simulink model "Simulation_04"  (R2014a)
settings: Solver=ode45  StartTime=0.0  StopTime=10.0  RelTol=1e-3
undefined symbols (not defined in the file or in its folder): sigbuilder_block
libraries: powerlib x12, simulink x1, powerlib_meascontrol x1
settings Model: Creator=Dell  LastModifiedBy=Dell

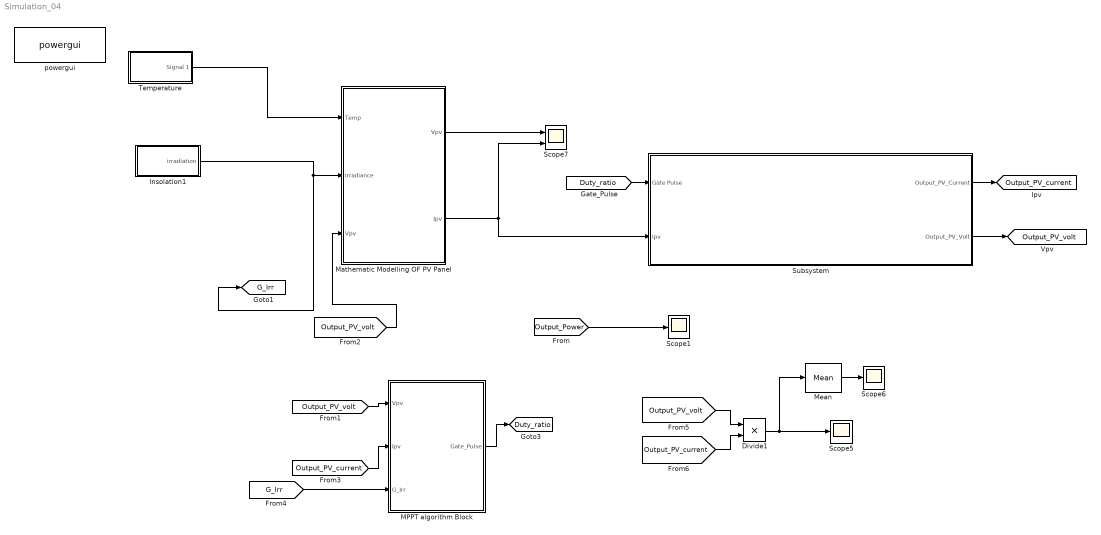
== system Simulation_04 ==
  Divide1 : Product  Inputs=**
  Insolation1 : Subsystem  Tag=STV Subsys  LoadFcn=sigbuilder_block('load');  StartFcn=sigbuilder_block('start');  StopFcn=sigbuilder_block('stop');  ClipboardFcn=sigbuilder_block('clipboard');  mask(Sigbuilder block){}
      mask help: Simulink:masks:SigbuilderBlock_MD
      mask init:
      | if ~strcmp(get_param(bdroot(gcbh),'SimulationStatus'),'stopped') tuvar = sigbuilder_block('maskInit'); end
      settings: CopyFcn=sigbuilder_block('copy');  DeleteFcn=sigbuilder_block('delete');  ModelCloseFcn=sigbuilder_block('modelClose');  PreSaveFcn=sigbuilder_block('preSave');  PauseFcn=sigbuilder_block('pause')  ContinueFcn=sigbuilder_block('continue')  NameChangeFcn=sigbuilder_block('namechange');  OpenFcn=sigbuilder_block('open',[557.25 17.25 550.5 394.5 ]);  CloseFcn=sigbuilder_block('close');
      mask Display: plot(0, 0, 100, 100,[2, 2, 32, 32, 2], [68, 8, 8, 68, 68],[32, 2], [38, 38], [32, 19, 2],[53, 60, 44], [32, 17, 17, 2],[16, 16, 31, 31]);txt = getActiveGroup(gcbh);text(2, 100, txt,'verticalAlignment', 'top');
  MPPT algorithm Block : Subsystem
  Mathematic Modelling OF PV Panel : Subsystem
      mask Display:
      | plot([0.3 0.4],[0.4 0.8]);
      | plot([0.4 0.5],[0.4 0.8]);
      | plot([0.5 0.6],[0.4 0.8]);
      | plot([0.6 0.7],[0.4 0.8]);
      | plot([0.3 0.6],[0.4 0.4]);
      | plot([0.325 0.625],[0.5 0.5]);
      | plot([0.35 0.65],[0.6 0.6]);
      | plot([0.375 0.675],[0.7 0.7]);
      | plot([0.4 0.7],[0.8 0.8]);
      | text(0.52,0.75,'PV module (V)','horizontalAlignment', 'center');
  Mean : powerlib_meascontrol/Measurements/Mean  Freq=60  Vinit=0  Ts=0
  Scope1 : Scope
      settings: TimeRange=2  YMin=220  YMax=252.5  SaveName=ScopeData2
  Scope5 : Scope
      settings: TimeRange=0.8  YMin=222.5  YMax=262.5  SaveName=ScopeData6
  Scope6 : Scope
      settings: TimeRange=0.8  YMin=258.52  YMax=258.65  SaveName=ScopeData7
  Scope7 : Scope  NumInputPorts=2
      settings: YMin=-22.5~7.325  YMax=35~7.6
  Subsystem : Subsystem
  Temperature : Subsystem  Tag=STV Subsys  LoadFcn=sigbuilder_block('load');  StartFcn=sigbuilder_block('start');  StopFcn=sigbuilder_block('stop');  ClipboardFcn=sigbuilder_block('clipboard');  mask(Sigbuilder block){}
      mask help: Simulink:masks:SigbuilderBlock_MD
      mask init:
      | if ~strcmp(get_param(bdroot(gcbh),'SimulationStatus'),'stopped') tuvar = sigbuilder_block('maskInit'); end
      settings: CopyFcn=sigbuilder_block('copy');  DeleteFcn=sigbuilder_block('delete');  ModelCloseFcn=sigbuilder_block('modelClose');  PreSaveFcn=sigbuilder_block('preSave');  PauseFcn=sigbuilder_block('pause');  ContinueFcn=sigbuilder_block('continue');  NameChangeFcn=sigbuilder_block('namechange');  OpenFcn=sigbuilder_block('open',[437.25 180 550.5 395.25 ]);  CloseFcn=sigbuilder_block('close');
      mask Display: plot(0, 0, 100, 100,[2, 2, 32, 32, 2], [68, 8, 8, 68, 68],[32, 2], [38, 38], [32, 19, 2],[53, 60, 44], [32, 17, 17, 2],[16, 16, 31, 31]);txt = getActiveGroup(gcbh);text(2, 100, txt,'verticalAlignment', 'top');
  powergui : powerlib/powergui  Priority=1  SimulationMode=Discrete  SolverType=Tustin  SampleTime=1e-6  frequency=60  SPID=off  DisableSnubberDevices=off  DisableRonSwitches=off  DisableVfSwitches=off  SwTol=0  Interpol=off  DisplayEquations=off  Ts=0  methode=off  frequencyindice=0  Pbase=100e6  ErrMax=1e-4  Iterations=50  UnitsV=kV  UnitsW=MW  FunctionMessages=off  echomessages=off  HookPort=off  EnableUseOfTLC=off  x0status=blocks  RestoreLinks=warning  ResistiveCurrentMeasurement=off  Frange=[0:2:500]  Ylog=off  Xlog=on  ShowGrid=off  save=off  variable=ZData  structure=0  ZoomFFT=off  StartTime=0.0  cycles=1  DisplayStyle=1  fundamental=60  FreqAxis=off  MaxFrequency=1000  frequencyindicesteady=1  RmsSteady=1  display=off
  tag scope: Duty_ratio=global, G_Irr=global, Output_PV_current=global, Output_PV_volt=global
  wires:
  [Output_Power] -> Scope1/1
  [Output_PV_volt] -> Divide1/1
  [Output_PV_current] -> Divide1/2
  Divide1/1 -> Scope5/1, Mean/1
  Mean/1 -> Scope6/1
  Temperature/1(Signal 1) -> Mathematic Modelling OF PV Panel/1(Temp)
  Insolation1/1(irradiation) -> [G_Irr], Mathematic Modelling OF PV Panel/2(Irradiance)
  Mathematic Modelling OF PV Panel/2(Ipv) -> Subsystem/2(Ipv), Scope7/2
  [Output_PV_volt] -> Mathematic Modelling OF PV Panel/3(Vpv)
  [Duty_ratio] -> Subsystem/1(Gate Pulse)
  Subsystem/1(Output_PV_Current) -> [Output_PV_current]
  Subsystem/2(Output_PV_Volt) -> [Output_PV_volt]
  [Output_PV_volt] -> MPPT algorithm Block/1(Vpv)
  [Output_PV_current] -> MPPT algorithm Block/2(Ipv)
  MPPT algorithm Block/1("Gate_Pulse ") -> [Duty_ratio]
  Mathematic Modelling OF PV Panel/1("Vpv ") -> Scope7/1
  [G_Irr] -> MPPT algorithm Block/3(G_Irr)

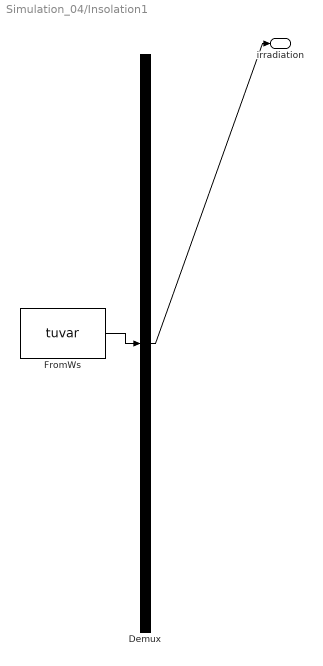
== system Simulation_04/Insolation1 ==
  Demux : Demux  Tag=STV Demux  Outputs=1
  FromWs : FromWorkspace  Tag=STV FromWs  VariableName=tuvar  SampleTime=0
      SigBuilderData=|
      | common.afterFinalStr = 'Extrapolate'
      | common.sampleTime = 0
      | dataSet.timeRange = [0 6]
      | dataSet.name = 'Group 1'
      | sbobj.Groups.Name = 'Group 1'
      | sbobj.Groups.Signals.Name = 'irradiation'
      | sbobj.Groups.Signals.XData = [0 2 3.99 4 6]
      | sbobj.Groups.Signals.YData = [1 1 1 1 1]
  irradiation : Outport  Tag=STV Outport
  wires:
  FromWs/1 -> Demux/1
  Demux/1 -> irradiation/1

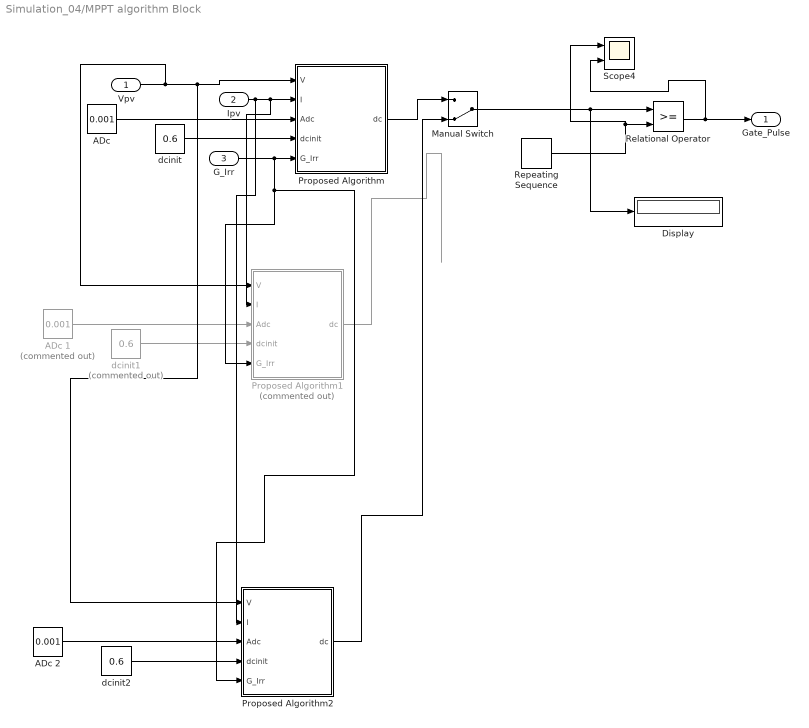
== system Simulation_04/MPPT algorithm Block ==
  Vpv : Inport
  Ipv : Inport  Port=2
  G_Irr : Inport  Port=3
  "ADc\t" : Constant  Value=0.001
  ADc	1 : Constant  Commented=on  Value=0.001
  ADc	2 : Constant  Value=0.001
  Display : Display
  Manual Switch : ManualSwitch  CurrentSetting=0
  Proposed Algorithm : MATLAB Function  TreatAsAtomicUnit=on
  Proposed Algorithm1 : MATLAB Function  Commented=on  TreatAsAtomicUnit=on
  Proposed Algorithm2 : MATLAB Function  TreatAsAtomicUnit=on
  Relational Operator : RelationalOperator  OutDataTypeStr=boolean
  Repeating Sequence : simulink/Sources/Repeating Sequence  rep_seq_t=[0 1/40000 1/20000]  rep_seq_y=[0 1 0]
  Scope4 : Scope  NumInputPorts=2
      settings: YMin=0~0  YMax=1~1  SaveName=ScopeData5
  dcinit : Constant  Value=0.6
  dcinit1 : Constant  Commented=on  Value=0.6
  dcinit2 : Constant  Value=0.6
  "Gate_Pulse " : Outport
  wires:
  Relational Operator/1 -> "Gate_Pulse "/1, Scope4/2
  Repeating Sequence/1 -> Scope4/1, Relational Operator/2
  dcinit/1 -> Proposed Algorithm/4(dcinit)
  "ADc\t"/1 -> Proposed Algorithm/3(Adc)
  dcinit1/1 -> Proposed Algorithm1/4(dcinit)
  ADc	1/1 -> Proposed Algorithm1/3(Adc)
  Proposed Algorithm/1(dc) -> Manual Switch/1
  Proposed Algorithm1/1(dc) -> ?
  Manual Switch/1 -> Display/1, Relational Operator/1
  Ipv/1 -> Proposed Algorithm2/2(I), Proposed Algorithm1/2(I), Proposed Algorithm/2(I)
  Vpv/1 -> Proposed Algorithm2/1(V), Proposed Algorithm/1(V), Proposed Algorithm1/1(V)
  dcinit2/1 -> Proposed Algorithm2/4(dcinit)
  ADc	2/1 -> Proposed Algorithm2/3(Adc)
  G_Irr/1 -> Proposed Algorithm2/5(G_Irr), Proposed Algorithm1/5(G_Irr), Proposed Algorithm/5(G_Irr)
  Proposed Algorithm2/1(dc) -> Manual Switch/2

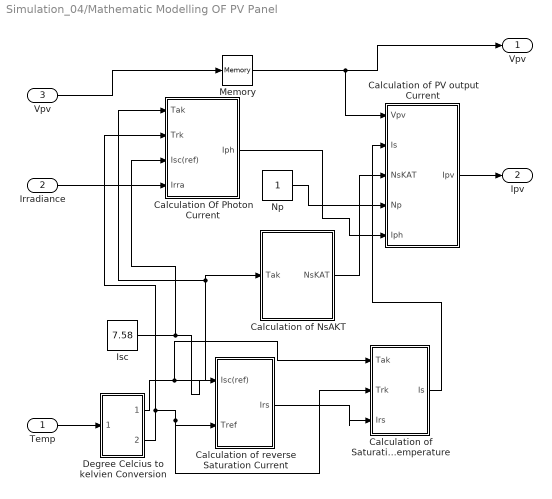
== system Simulation_04/Mathematic Modelling OF PV Panel ==
  Temp : Inport
  Irradiance : Inport  Port=2
  Vpv : Inport  Port=3
  "Calculation Of Photon Current " : Subsystem
  Calculation of Saturation Current Varies With Temperature : Subsystem
  Calculation of NsAKT : Subsystem
  "Calculation of PV output Current " : Subsystem
  Calculation of reverse Saturation Current : Subsystem
  Degree Celcius to kelvien Conversion : Subsystem
  Isc : Constant  Value=7.58
  Memory : Memory
  Np : Constant
  "Vpv " : Outport
  Ipv : Outport  Port=2
  wires:
  Calculation of Saturation Current Varies With Temperature/1(Is) -> "Calculation of PV output Current "/2(Is)
  Calculation of reverse Saturation Current/1(Irs) -> Calculation of Saturation Current Varies With Temperature/3("Irs ")
  Np/1 -> "Calculation of PV output Current "/4(Np)
  Temp/1 -> Degree Celcius to kelvien Conversion/1("Top ")
  "Calculation of PV output Current "/1("Ipv ") -> Ipv/1
  Irradiance/1 -> "Calculation Of Photon Current "/4(Irra)
  Degree Celcius to kelvien Conversion/1(Tak) -> Calculation of Saturation Current Varies With Temperature/1(Tak), "Calculation Of Photon Current "/1(Tak), Calculation of NsAKT/1("Tak ")
  "Calculation Of Photon Current "/1(Iph) -> "Calculation of PV output Current "/5(Iph)
  Calculation of NsAKT/1(NsKAT) -> "Calculation of PV output Current "/3(NsKAT)
  Isc/1 -> "Calculation Of Photon Current "/3(Isc(ref)), Calculation of reverse Saturation Current/1("Isc(ref) ")
  Degree Celcius to kelvien Conversion/2(Trk) -> "Calculation Of Photon Current "/2(Trk), Calculation of Saturation Current Varies With Temperature/2("Trk "), Calculation of reverse Saturation Current/2("Tref ")
  Vpv/1 -> Memory/1
  Memory/1 -> "Calculation of PV output Current "/1(Vpv), "Vpv "/1

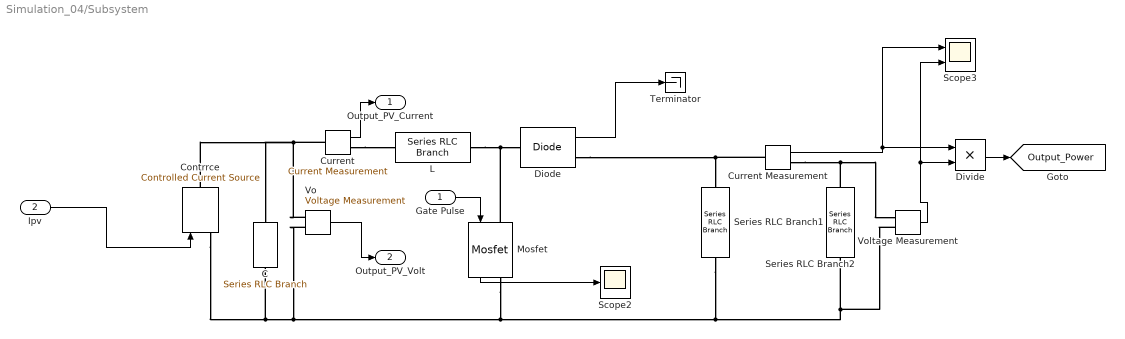
== system Simulation_04/Subsystem ==
  Gate Pulse : Inport
  Ipv : Inport  Port=2
  C : powerlib/Elements/Series RLC Branch  LConnTagsString=__new0  RConnTagsString=__new0  BranchType=C  Resistance=10  Inductance=5e-3  SetiL0=on  InitialCurrent=0  Capacitance=1e-6  Setx0=off  InitialVoltage=0  Measurements=None
  Contrrce : powerlib/Electrical Sources/Controlled Current Source  Initialize=on  Source_Type=DC  Amplitude=0  Phase=0  Frequency=0  Measurements=None
  "Current " : powerlib/Measurements/Current Measurement  PhasorSimulation=off  OutputType=Complex  PSBequivalent=0
  Current Measurement : powerlib/Measurements/Current Measurement  PhasorSimulation=off  OutputType=Complex  PSBequivalent=0
  Diode : powerlib/Power Electronics/Diode  Ron=0.001  Lon=0  Vf=0.8  IC=0  UseSnubber=off  Rs=500*0  Cs=250e-9*0  Measurements=on
  Divide : Product  Inputs=**
  L : powerlib/Elements/Series RLC Branch  LConnTagsString=__new0  RConnTagsString=__new0  BranchType=L  Resistance=10  Inductance=5e-3  SetiL0=on  InitialCurrent=0  Capacitance=1e-6  Setx0=off  InitialVoltage=0  Measurements=None
  Mosfet : powerlib/Power Electronics/Mosfet  Ron=0.1  Lon=0  Rd=0.01  Vfd=0  IC=0  Rs=1e5  Cs=inf  Measurements=on
  Scope2 : Scope
      settings: YMin=-5.49725  YMax=49.47525  SaveName=ScopeData3
  Scope3 : Scope  NumInputPorts=2
      settings: YMin=2.52~100.8  YMax=2.536~101.45  SaveName=ScopeData4
  Series RLC Branch1 : powerlib/Elements/Series RLC Branch  LConnTagsString=__new0  RConnTagsString=__new0  BranchType=C  Resistance=1  Inductance=5e-3  SetiL0=on  InitialCurrent=0  Capacitance=270e-6  Setx0=on  InitialVoltage=0  Measurements=None
  Series RLC Branch2 : powerlib/Elements/Series RLC Branch  LConnTagsString=__new0  RConnTagsString=__new0  BranchType=R  Resistance=60  Inductance=5e-3  SetiL0=on  InitialCurrent=0  Capacitance=1e-6  Setx0=off  InitialVoltage=0  Measurements=None
  Terminator : Terminator
  Vo : powerlib/Measurements/Voltage Measurement  PhasorSimulation=off  OutputType=Complex  PSBequivalent=0
  Voltage Measurement : powerlib/Measurements/Voltage Measurement  PhasorSimulation=off  OutputType=Complex  PSBequivalent=0
  Output_PV_Current : Outport
  Output_PV_Volt : Outport  Port=2
  tag scope: Output_Power=global
  wires:
  Ipv/1 -> Contrrce/1
  Diode/1 -> Terminator/1
  Divide/1 -> [Output_Power]
  Voltage Measurement/1 -> Scope3/2, Divide/2
  Vo/1 -> Output_PV_Volt/1
  Gate Pulse/1 -> Mosfet/1
  "Current "/1 -> Output_PV_Current/1
  Current Measurement/1 -> Divide/1, Scope3/1
  Mosfet/1 -> Scope2/1
  connections:
  Diode/RConn1 -- Current Measurement/LConn1 -- Series RLC Branch1/LConn1
  Vo/LConn1 -- Contrrce/RConn1 -- C/LConn1 -- "Current "/LConn1
  Series RLC Branch2/LConn1 -- Current Measurement/RConn1 -- Voltage Measurement/LConn1
  Contrrce/LConn1 -- C/RConn1 -- Vo/LConn2 -- Mosfet/RConn1 -- Series RLC Branch1/RConn1 -- Voltage Measurement/LConn2 -- Series RLC Branch2/RConn1
  "Current "/RConn1 -- L/LConn1
  L/RConn1 -- Mosfet/LConn1 -- Diode/LConn1

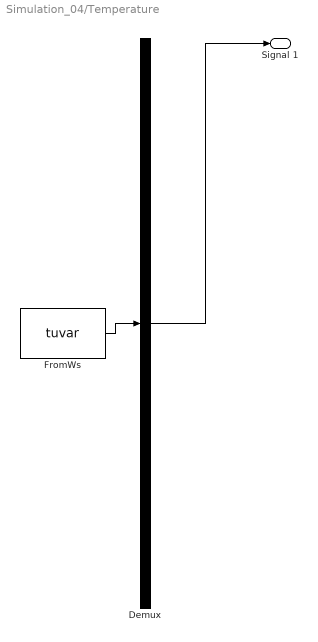
== system Simulation_04/Temperature ==
  Demux : Demux  Tag=STV Demux  Outputs=1
  FromWs : FromWorkspace  Tag=STV FromWs  VariableName=tuvar  SampleTime=0
      SigBuilderData=|
      | common.afterFinalStr = 'Extrapolate'
      | common.sampleTime = 0
      | dataSet.timeRange = [0 10]
      | dataSet.name = 'Group 1'
      | sbobj.Groups.Name = 'Group 1'
      | sbobj.Groups.Signals.Name = 'Signal 1'
      | sbobj.Groups.Signals.XData = [0 2 4 10]
      | sbobj.Groups.Signals.YData = [25 25 25 25]
  Signal 1 : Outport  Tag=STV Outport
  wires:
  Demux/1 -> Signal 1/1
  FromWs/1 -> Demux/1

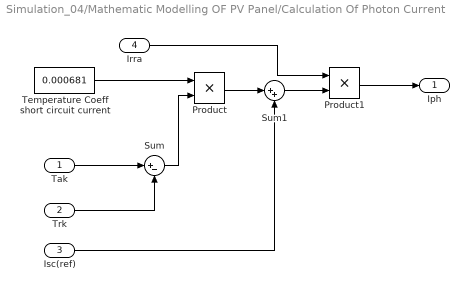
== system Simulation_04/Mathematic Modelling OF PV Panel/Calculation Of Photon Current  ==
  Tak : Inport
  Trk : Inport  Port=2
  Isc(ref) : Inport  Port=3
  Irra : Inport  Port=4
  Product : Product
  Product1 : Product
  Sum : Sum  Inputs=|+-
  Sum1 : Sum  Inputs=|++
  "Temperature Coeff short circuit current " : Constant  Value=0.000681
  Iph : Outport
  wires:
  Product/1 -> Sum1/1
  Trk/1 -> Sum/2
  "Temperature Coeff short circuit current "/1 -> Product/1
  Irra/1 -> Product1/1
  Isc(ref)/1 -> Sum1/2
  Tak/1 -> Sum/1
  Sum1/1 -> Product1/2
  Sum/1 -> Product/2
  Product1/1 -> Iph/1

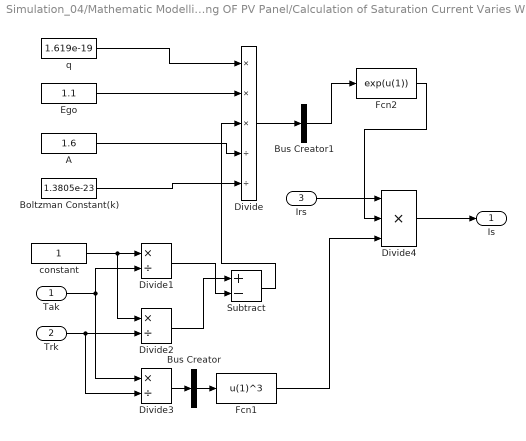
== system Simulation_04/Mathematic Modelling OF PV Panel/Calculation of Saturation Current Varies With Temperature ==
  Tak : Inport
  "Trk " : Inport  Port=2
  "Irs " : Inport  Port=3
  "A " : Constant  Value=1.6
  Boltzman Constant(k) : Constant  Value=1.3805e-23
  Bus Creator : BusCreator  Inputs=1
  Bus Creator1 : BusCreator  Inputs=1
  Divide : Product  Inputs=***//
  Divide1 : Product  Inputs=*/
  Divide2 : Product  Inputs=*/
  Divide3 : Product  Inputs=*/
  Divide4 : Product  Inputs=***
  Ego : Constant  Value=1.1
  Fcn1 : Fcn  Expr=u(1)^3
  Fcn2 : Fcn  Expr=exp(u(1))
  Subtract : Sum  Inputs=+-
  "constant " : Constant
  "q " : Constant  Value=1.619e-19
  Is : Outport
  wires:
  "constant "/1 -> Divide2/1, Divide1/1
  Bus Creator1/1 -> Fcn2/1
  Divide/1 -> Bus Creator1/1
  Divide1/1 -> Subtract/2
  Fcn1/1 -> Divide4/3
  Divide2/1 -> Subtract/1
  Tak/1 -> Divide1/2, Divide3/1
  Fcn2/1 -> Divide4/2
  "Trk "/1 -> Divide3/2, Divide2/2
  "A "/1 -> Divide/4
  Ego/1 -> Divide/2
  Subtract/1 -> Divide/3
  Boltzman Constant(k)/1 -> Divide/5
  "q "/1 -> Divide/1
  "Irs "/1 -> Divide4/1
  Divide4/1 -> Is/1
  Bus Creator/1 -> Fcn1/1
  Divide3/1 -> Bus Creator/1

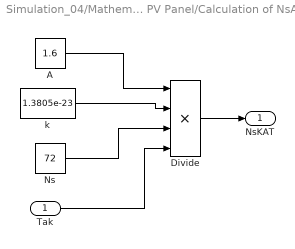
== system Simulation_04/Mathematic Modelling OF PV Panel/Calculation of NsAKT ==
  "Tak " : Inport
  A : Constant  Value=1.6
  Divide : Product  Inputs=****
  Ns : Constant  Value=72
  k : Constant  Value=1.3805e-23
  NsKAT : Outport
  wires:
  Ns/1 -> Divide/3
  A/1 -> Divide/1
  k/1 -> Divide/2
  "Tak "/1 -> Divide/4
  Divide/1 -> NsKAT/1

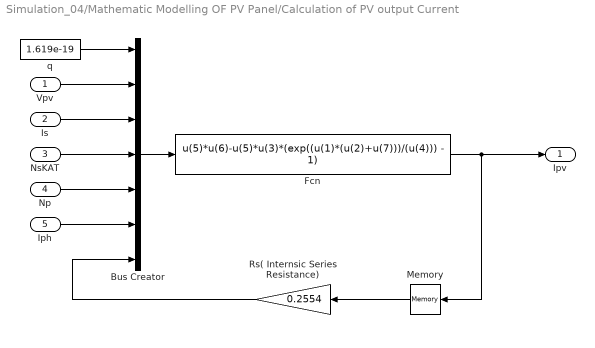
== system Simulation_04/Mathematic Modelling OF PV Panel/Calculation of PV output Current  ==
  Vpv : Inport
  Is : Inport  Port=2
  NsKAT : Inport  Port=3
  Np : Inport  Port=4
  Iph : Inport  Port=5
  Bus Creator : BusCreator  Inputs=7
  Fcn : Fcn  Expr=u(5)*u(6)-u(5)*u(3)*(exp((u(1)*(u(2)+u(7)))/(u(4))) - 1)
  Memory : Memory
  Rs( Internsic Series Resistance) : Gain  Gain=0.2554
  q : Constant  Value=1.619e-19
  "Ipv " : Outport
  wires:
  Vpv/1 -> Bus Creator/2
  Is/1 -> Bus Creator/3
  Fcn/1 -> Memory/1, "Ipv "/1
  Bus Creator/1 -> Fcn/1
  Rs( Internsic Series Resistance)/1 -> Bus Creator/7
  Iph/1 -> Bus Creator/6
  Np/1 -> Bus Creator/5
  q/1 -> Bus Creator/1
  NsKAT/1 -> Bus Creator/4
  Memory/1 -> Rs( Internsic Series Resistance)/1

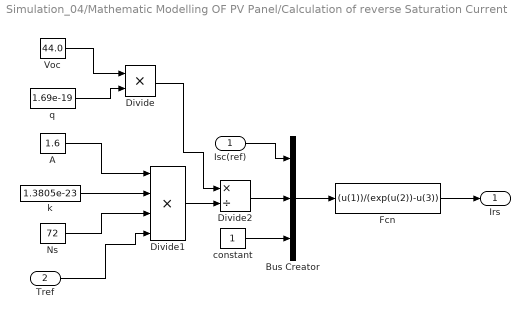
== system Simulation_04/Mathematic Modelling OF PV Panel/Calculation of reverse Saturation Current ==
  "Isc(ref) " : Inport
  "Tref " : Inport  Port=2
  A : Constant  Value=1.6
  Bus Creator : BusCreator  Inputs=3
  Divide : Product  Inputs=**
  Divide1 : Product  Inputs=****
  Divide2 : Product  Inputs=*/
  Fcn : Fcn  Expr=(u(1))/(exp(u(2))-u(3))
  Ns : Constant  Value=72
  Voc : Constant  Value=44.0
  "constant " : Constant
  k : Constant  Value=1.3805e-23
  q : Constant  Value=1.69e-19
  Irs : Outport
  wires:
  Voc/1 -> Divide/1
  Divide/1 -> Divide2/1
  k/1 -> Divide1/2
  "constant "/1 -> Bus Creator/3
  Divide2/1 -> Bus Creator/2
  Bus Creator/1 -> Fcn/1
  "Tref "/1 -> Divide1/4
  Fcn/1 -> Irs/1
  q/1 -> Divide/2
  A/1 -> Divide1/1
  "Isc(ref) "/1 -> Bus Creator/1
  Ns/1 -> Divide1/3
  Divide1/1 -> Divide2/2

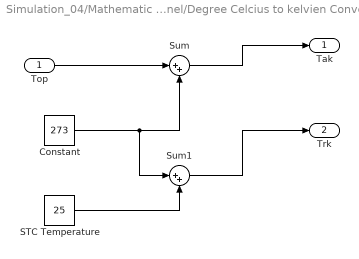
== system Simulation_04/Mathematic Modelling OF PV Panel/Degree Celcius to kelvien Conversion ==
  "Top " : Inport
  Constant : Constant  Value=273
  STC Temperature : Constant  Value=25
  Sum : Sum  Inputs=|++
  Sum1 : Sum  Inputs=|++
  Tak : Outport
  Trk : Outport  Port=2
  wires:
  Sum1/1 -> Trk/1
  Constant/1 -> Sum1/1, Sum/2
  "Top "/1 -> Sum/1
  Sum/1 -> Tak/1
  STC Temperature/1 -> Sum1/2

== matlab function Simulation_04/MPPT algorithm Block/Proposed Algorithm1 ==
  data: V input; dc output; I input; Adc input; dcinit input; G_Irr input
function dc = IC( V, I, Adc, dcinit, G_Irr)

 
% persistent dco Vo Io
% dataType = 'double';
%    
%             if isempty(Vo)
%                 Vo=0;
%                 Io=0;
%                 dco=dcinit;
%             end
% 
%           
%             dV=V-Vo;
%             dI=I-Io;
%           
%             if dV==0
%                 if dI==0
%                     dc =dco;
%                     return
%                 else
%                     if dI>0
%                         dc = dco + Adc; 
%                     else
%                         dc = dco - Adc; 
%                     end
%                 end
%             else
%                 if I+(dI/dV)*V==0
%                     dc=dco;
%                     return
%                 else
%                     if I+(dI/dV)*V>0
%                         dc = dco - Adc; 
%                     else
%                         dc = dco + Adc; 
%                     end
%                 end
%             end
%             dcmax=0.95; 
%               dcmin=0.05;
%             if dc>=dcmax || dc<=dcmin
%                 dc=dco;
%             end
% 
%             dco=dc;
%             Vo=V;
%             Io=I;
%      
persistent dmp Vo Io
dataType = 'double';
        
            if isempty(Vo)
             dmp=0.711;
             Vo=zeros(3,1);
             Io=zeros(3,1);
            end
            
            dc=dmp;
            Vo(1)=36.2;
            Io(1)=7.1;
            
          for i=2:3  
            if dc==0.69
                 dc=dmp -0.2*dmp;
                 Vo(i)=V;
                 Io(i)=I;
                 

 
 
  
     end

== matlab function Simulation_04/MPPT algorithm Block/Proposed Algorithm2 ==
  data: V input; dc output; I input; Adc input; dcinit input; G_Irr input
function dc = IC( V, I, Adc, dcinit, G_Irr)

persistent dco Vo Io
dataType= 'double';

            
            dco=0.711;
            Vo=zeros(3,1);
            Io=zeros(3,1);
            dc=dco;
            
if dco==0.711
       dc=dco + 0.2*dco;
else
    dc=dco;
end


end



 
% persistent dco Vo Io
% dataType = 'double';
%    
%             if isempty(Vo)
%                 Vo=0;
%                 Io=0;
%                 dco=dcinit;
%             end
% 
%           
%             dV=V-Vo;
%             dI=I-Io;
%           
%             if dV==0
%                 if dI==0
%                     dc =dco;
%                     return
%                 else
%                     if dI>0
%                         dc = dco + Adc; 
%                     else
%                         dc = dco - Adc; 
%                     end
%                 end
%             else
%                 if I+(dI/dV)*V==0
%                     dc=dco;
%                     return
%                 else
%                     if I+(dI/dV)*V>0
%                         dc = dco - Adc; 
%                     else
%                         dc = dco + Adc; 
%                     end
%                 end
%             end
%             dcmax=0.95; 
%               dcmin=0.05;
%             if dc>=dcmax || dc<=dcmin
%                 dc=dco;
%             end
% 
%             dco=dc;
%             Vo=V;
%             Io=I;
%      
% persistent dmp Vo Io
% dataType = 'double';
%         
%             if isempty(Vo)
%              dmp=0.711;
%              Vo=zeros(3,1);
%              Io=zeros(3,1);
%             end
%             
%             dc=dmp;
%             Vo(1)=36.2;
%             Io(1)=7.1;
%             
%           for i=2:3  
%             if dc==0.69
%                  dc=dmp -0.2*dmp;
%                  Vo(i)=V;
%                  Io(i)=I;
%

== matlab function Simulation_04/MPPT algorithm Block/Proposed Algorithm ==
  data: V input; dc output; I input; Adc input; dcinit input; G_Irr input
function dc = IC( V, I, Adc, dcinit, G_Irr)


persistent dco Vo Io
dataType = 'double';
   
            if isempty(Vo)
                Vo=0;
                Io=0;
                dco=dcinit;
            end

          
            dV=V-Vo;
            dI=I-Io;
          
            if dV==0
                if dI==0
                    dc =dco;
                    return
                else
                    if dI>0
                        dc = dco + Adc; 
                    else
                        dc = dco - Adc; 
                    end
                end
            else
                if I+(dI/dV)*V==0
                    dc=dco;
                    return
                else
                    if I+(dI/dV)*V>0
                        dc = dco - Adc; 
                    else
                        dc = dco + Adc; 
                    end
                end
            end
            dcmax=0.95; 
              dcmin=0.05;
            if dc>=dcmax || dc<=dcmin
                dc=dco;
            end

            dco=dc;
            Vo=V;
            Io=I;
     
         
     end
